simulink model "Multi_Quad"  (R2025b)
settings: Solver=ode4  StartTime=0.0  StopTime=80.0  FixedStep=0.001  RelTol=1e-3
values from neighbouring files (symbols this model uses):
  D = zeros(num_agents, num_agents)    [init_multi.m]
  d0 = zeros(num_agents, 1)    [init_multi.m]
  delta = zeros(3, 4)    [init_multi.m]    (also in init_single.m = [1; 1; 0]; plot_multi.m; plot_single.m = [1; 1; 0])
  g = 9.81    [init_multi.m]    (also in init_single.m)
  J = diag([0.04856, 0.04856, 0.08801])    [init_multi.m]    (also in init_single.m = diag([J_xx, J_yy, J_zz]))
  k_rho = 0.5    [init_multi.m]    (also in init_single.m)
  ka = 30    [init_multi.m]
  kp = 3    [init_multi.m]    (also in init_single.m)
  kq = 16    [init_multi.m]
  kt = 20    [init_multi.m]    (also in init_single.m)
  kv = 3    [init_multi.m]    (also in init_single.m)
  kw = 3    [init_multi.m]    (also in init_single.m)
  m = 1    [init_multi.m]    (also in init_single.m)
  xInitial = [p0_all; v0_all; Q0_all; w0_all]    [init_multi.m]
settings Model: Creator=ZhuanZ（无密码）  LastModifiedBy=ZhuanZ（无密码）
settings DataIOCC: ReturnWorkspaceOutputs=off

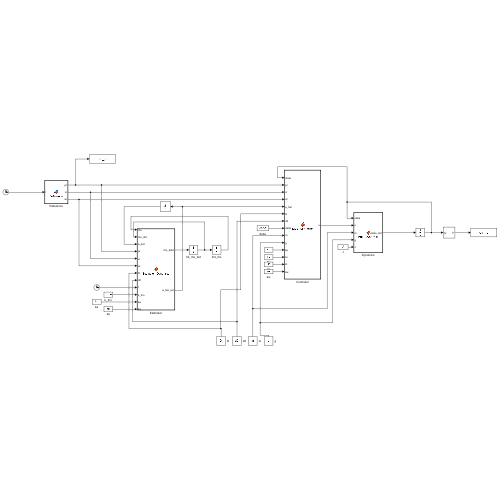
[thumbnail: Simulink's stored preview of the top-level diagram]
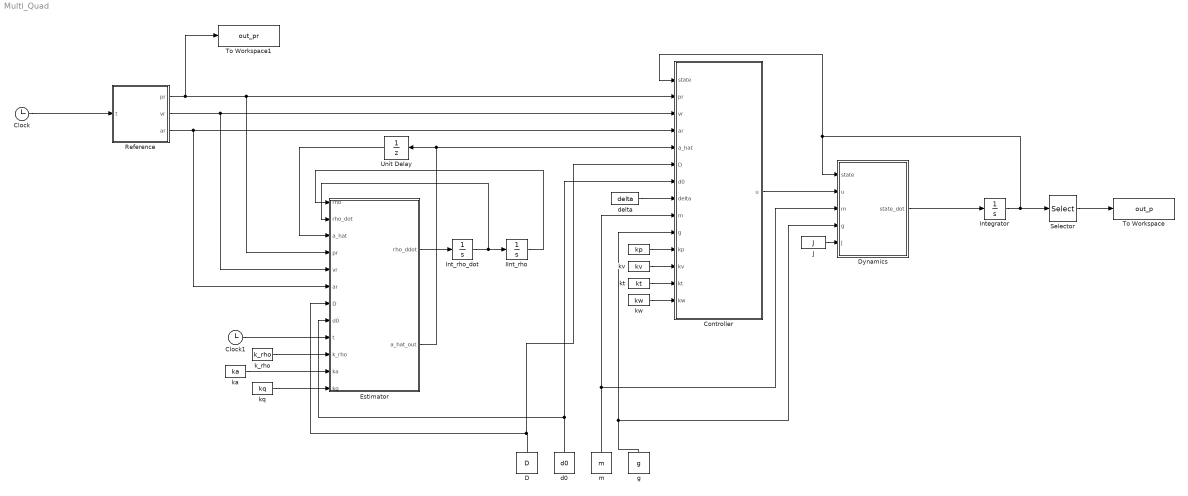
== system Multi_Quad ==
  " " : Constant  Value=kp
  Clock : Clock
  Clock1 : Clock
  Controller : MATLAB Function  TreatAsAtomicUnit=on
  D : Constant  Value=D
  Dynamics : MATLAB Function  TreatAsAtomicUnit=on
  Estimator : MATLAB Function  TreatAsAtomicUnit=on
  IInt_rho : Integrator
  Int_rho_dot : Integrator
  Integrator : Integrator  InitialCondition=xInitial
  J : Constant  Value=J
  Reference : MATLAB Function  TreatAsAtomicUnit=on
  Selector : Selector  NumberOfDimensions=2  InputPortWidth=13  IndexOptions=Index vector (dialog),Select all  Indices=[1 2 3],1  OutputSizes=1,1
  To Workspace : ToWorkspace  VariableName=out_p  SaveFormat=Timeseries  SampleTime=-1
  To Workspace1 : ToWorkspace  VariableName=out_pr  SaveFormat=Timeseries  SampleTime=-1
  Unit Delay : UnitDelay  InitialCondition=zeros(3,4)  SampleTime=-1  HasFrameUpgradeWarning=on
  d0 : Constant  Value=d0
  delta : Constant  Value=delta
  g : Constant  Value=g
  k_rho : Constant  Value=k_rho
  ka : Constant  Value=ka  VectorParams1D=off
  kq : Constant  Value=kq
  kt : Constant  Value=kt
  kv : Constant  Value=kv
  kw : Constant  Value=kw
  m : Constant  Value=m
  wires:
  Clock/1 -> Reference/1(t)
  Reference/3(ar) -> Estimator/6(ar), Controller/4(ar)
  Reference/2(vr) -> Estimator/5(vr), Controller/3(vr)
  Reference/1(pr) -> To Workspace1/1, Estimator/4(pr), Controller/2(pr)
  Controller/1(u) -> Dynamics/2(u)
  Dynamics/1(state_dot) -> Integrator/1
  Integrator/1 -> Dynamics/1(state), Controller/1(state), Selector/1
  Selector/1 -> To Workspace/1
  Estimator/1(rho_ddot) -> Int_rho_dot/1
  Int_rho_dot/1 -> Estimator/2(rho_dot), IInt_rho/1
  IInt_rho/1 -> Estimator/1(rho)
  Clock1/1 -> Estimator/9(t)
  k_rho/1 -> Estimator/10(k_rho)
  kq/1 -> Estimator/12(kq)
  ka/1 -> Estimator/11(ka)
  D/1 -> Controller/6(D), Estimator/7(D)
  d0/1 -> Controller/7(d0), Estimator/8(d0)
  m/1 -> Dynamics/3(m), Controller/9(m)
  delta/1 -> Controller/8(delta)
  g/1 -> Dynamics/4(g), Controller/10(g)
  J/1 -> Dynamics/5(J)
  " "/1 -> Controller/11(kp)
  kv/1 -> Controller/12(kv)
  kt/1 -> Controller/13(kt)
  kw/1 -> Controller/14(kw)
  Estimator/2(a_hat_out) -> Controller/5(a_hat), Unit Delay/1
  Unit Delay/1 -> Estimator/3(a_hat)

== matlab function Multi_Quad/Controller ==
  data: state input; u output; pr input; vr input; ar input; a_hat input; D input; d0 input; delta input; m input; g input; kp input; kv input; kt input; kw input
function u = Multi_Controller(state, pr, vr, ar, a_hat, D, d0, delta, m, g, kp, kv, kt, kw)
    % 解包状态 (注意现在是矩阵)
    % p, v: 3x4
    % Q: 4x4
    % w: 3x4
    p = state(1:3, :);
    v = state(4:6, :);
    Q = state(7:10, :);
    w = state(11:13, :);
    
    num = 4;
    u = zeros(4, num); % 输出 [T; tau_x; tau_y; tau_z] x 4
    
    % 循环处理每一架飞机 (这是最稳妥的写法)
    for i = 1:num
        % --- 1. 位置环 (论文 Eq. 10) ---
        
        % 计算位置误差求和项 (P项)
        sum_pos_err = [0;0;0];
        for j = 1:num
            if D(i,j) > 0
                % 邻居误差: (pi - pj - delta_ij)
                % delta_ij = delta_i - delta_j
                delta_ij = delta(:,i) - delta(:,j);
                sum_pos_err = sum_pos_err + D(i,j) * (p(:,i) - p(:,j) - delta_ij);
            end
        end
        % 领航者误差: d_i0 * (pi - pr - delta_i)
        leader_pos_err = d0(i) * (p(:,i) - pr - delta(:,i));
        
        term_P = sum_pos_err + leader_pos_err;
        
        % 计算速度误差求和项 (V项)
        sum_vel_err = [0;0;0];
        for j = 1:num
            if D(i,j) > 0
                sum_vel_err = sum_vel_err + D(i,j) * (v(:,i) - v(:,j));
            end
        end
        leader_vel_err = d0(i) * (v(:,i) - vr);
        
        term_V = sum_vel_err + leader_vel_err;
        
        % 合成虚拟力 u_c (Eq. 10)
        % 注意：这里使用了 Estimator 传过来的 a_hat(:,i)
        e3 = [0;0;1];
        u_c = m * (g*e3 + a_hat(:,i) ...
                   - kp * tanh(term_P) ...
                   - kv * tanh(term_V));
                   
        % --- 2. 姿态提取 (Eq. 18) ---
        % (这部分和单机一样，只是包在循环里)
        norm_uc = norm(u_c);
        if norm_uc < 1e-6, norm_uc = 1e-6; end
        
        T = norm_uc; % 推力
        
        u_z = u_c(3);
        sigma_c = sqrt(0.5 * (1 + u_z/norm_uc));
        if sigma_c < 1e-6, sigma_c = 1e-6; end
        
        % 这里的叉乘方向依然保持你单机代码修正后的逻辑
        qc_vec = (1 / (2*norm_uc*sigma_c)) * [-u_c(2); u_c(1); 0];
        Qc = [sigma_c; qc_vec];
        
        % --- 3. 姿态环 (Eq. 24 简化版 PD) ---
        Q_curr = Q(:,i);
        w_curr = w(:,i);
        
        % 姿态误差
        Qc_inv = [Qc(1); -Qc(2:4)];
        Qe_sigma = Qc_inv(1)*Q_curr(1) - dot(Qc_inv(2:4), Q_curr(2:4));
        Qe_vec   = Qc_inv(1)*Q_curr(2:4) + Q_curr(1)*Qc_inv(2:4) + cross(Qc_inv(2:4), Q_curr(2:4));
        
        if Qe_sigma < 0
            Qe_vec = -Qe_vec;
        end
        
        tau = -kt * Qe_vec - kw * w_curr;
        
        % 打包输出
        u(:,i) = [T; tau];
    end
end

== matlab function Multi_Quad/Reference ==
  data: t input; pr output; vr output; ar output
function [pr, vr, ar] = Reference(t)
    % 论文 Section IV 的 8 字形螺旋轨迹
    % pr: 位置, vr: 速度, ar: 加速度
    
    % 位置 pr = [3cos(0.2t), 2sin(0.2t), t]
    pr = [3*cos(0.2*t); 2*sin(0.2*t); t];
    
    % 速度 (对时间求导)
    vr = [-0.6*sin(0.2*t); 0.4*cos(0.2*t); 1];
    
    % 加速度 (再求导)
    ar = [-0.12*cos(0.2*t); -0.08*sin(0.2*t); 0];
end

== matlab function Multi_Quad/Dynamics ==
  data: state input; u input; state_dot output; m input; g input; J input
function state_dot = Multi_Dynamics(state, u, m, g, J)
    % state: 13x4
    % u: 4x4
    
    num = 4;
    state_dot = zeros(13, num);
    e3 = [0;0;1];
    
    for i = 1:num
        % 提取单机状态
        p = state(1:3, i);
        v = state(4:6, i);
        Q = state(7:10, i);
        w = state(11:13, i);
        
        T = u(1, i);
        tau = u(2:4, i);
        
        % 1. 位置导数
        p_dot = v;
        
        % 2. 速度导数
        s = Q(1); x = Q(2); y = Q(3); z = Q(4);
        R = [1-2*(y^2+z^2), 2*(x*y-s*z),   2*(x*z+s*y);
             2*(x*y+s*z),   1-2*(x^2+z^2), 2*(y*z-s*x);
             2*(x*z-s*y),   2*(y*z+s*x),   1-2*(x^2+y^2)];
        
        v_dot = -g*e3 + (T/m) * R * e3;
        
        % 3. 四元数导数
        Q_dot = 0.5 * [ -x, -y, -z;
                         s, -z,  y;
                         z,  s, -x;
                        -y,  x,  s ] * w;
        
        % 4. 角速度导数
        w_dot = J \ (-cross(w, J*w) + tau);
        
        % 填入结果
        state_dot(:, i) = [p_dot; v_dot; Q_dot; w_dot];
    end
end

== matlab function Multi_Quad/Estimator ==
  data: rho input; rho_ddot output; rho_dot input; a_hat input; pr input; vr input; ar input; D input; d0 input; t input; k_rho input; ka input; kq input; a_hat_out output
function [rho_ddot, a_hat_out] = Estimator_Dynamics(rho, rho_dot, a_hat, pr, vr, ar, D, d0, t, k_rho, ka, kq)
    % 论文 Eq. 11: 分布式有限时间估计器
    % 处理 4 架无人机的矩阵运算
    
    num = 4;
    rho_ddot = zeros(3, num);
    a_hat_out = zeros(3, num); % 输出新的 a_hat 供控制器使用
    
    % 有限时间函数 epsilon(t) = exp(-0.5 * t)
    % 为了防止分母为0，加一个极小值
    eps_t = exp(-0.5 * t) + 1e-6; 
    
    % 领航者的 jerk (p_r的三阶导)。
    % 你的 Reference 代码里 ar 是 [-0.12*cos; ...]
    % 这里简单起见，假设 jerk = 0 (或者你可以去求导 Reference)
    % 论文里如果轨迹是缓慢变化的，这项影响不大。
    % 严谨的话，需要在 Reference 里增加 jerk 输出。
    jerk_r = zeros(3,1); 
    
    % 计算 a_hat (代数关系)
    for i = 1:num
        a_hat_out(:,i) = k_rho * tanh(rho(:,i));
    end
    
    % 计算 rho 的二阶导数 (Eq. 11)
    for i = 1:num
        % --- 准备求和项 ---
        sum_neighbors_1 = zeros(3,1); % sum d_ij (a_i - a_j)
        sum_neighbors_2 = zeros(3,1); % sum d_ij (a_dot_i - a_dot_j) -> 这里论文略有简略，其实可以用差分近似
        
        % 注意：Eq 11 里有 a_hat_dot。
        % 因为 a_hat = k * tanh(rho), 所以 a_hat_dot = k * sechk^2(rho) * rho_dot
        % 我们先算出当前时刻每架飞机的 a_hat_dot
        sech_sq = 1 - tanh(rho(:,i)).^2;
        a_hat_dot_i = k_rho * (sech_sq .* rho_dot(:,i));
        
        for j = 1:num
            if D(i,j) > 0
                % 邻居 j 的 a_hat_dot
                sech_sq_j = 1 - tanh(rho(:,j)).^2;
                a_hat_dot_j = k_rho * (sech_sq_j .* rho_dot(:,j));
                
                sum_neighbors_1 = sum_neighbors_1 + D(i,j) * (a_hat(:,i) - a_hat(:,j));
                sum_neighbors_2 = sum_neighbors_2 + D(i,j) * (a_hat_dot_i - a_hat_dot_j);
            end
        end
        
        % 领航者误差项
        leader_term_1 = d0(i) * (a_hat(:,i) - ar);      % (a_hat - p_r_ddot)
        leader_term_2 = d0(i) * (a_hat_dot_i - jerk_r); % (a_hat_dot - p_r_triple_dot)
        
        % 巨大的括号里的分子
        numerator = sum_neighbors_1 + leader_term_1;
        numerator_dot = sum_neighbors_2 + leader_term_2;
        
        % 论文中的 Xi_i 矩阵 (对角阵)
        % Xi = diag(tanh(rho)*rho_dot)
        Xi = rho_dot(:,i) .* tanh(rho(:,i)); % 简化写成向量形式
        
        % 论文中的 Upsilon_i 矩阵的逆
        % Upsilon = diag(1 - tanh^2)
        % Inv_Upsilon = 1 / (1 - tanh^2)
        inv_Upsilon = 1 ./ (1 - tanh(rho(:,i)).^2 + 1e-6); 
        
        % --- 核心公式 Eq. 11 ---
        % 第一行: (2*Xi - I) * rho_dot
        term1 = (2 * Xi - 1) .* rho_dot(:,i);
        
        % 第二行: Inverse * [ ... ]
        term_bracket = (kq/k_rho) * numerator + ...
                       (ka/k_rho) * tanh( (numerator/eps_t) + (numerator_dot/eps_t) );
                   
        rho_ddot(:,i) = term1 - inv_Upsilon .* term_bracket;
    end
end
